simulink model "sedemsegment"  (Simulink 7.7)
settings: Solver=ode45  StartTime=0.0  StopTime=1  RelTol=1e-3
libraries: simulink x18
settings Model: Creator=RIchard  LastModifiedBy=RIchard
settings DebuggingCC: SolverPrmCheckMsg=none

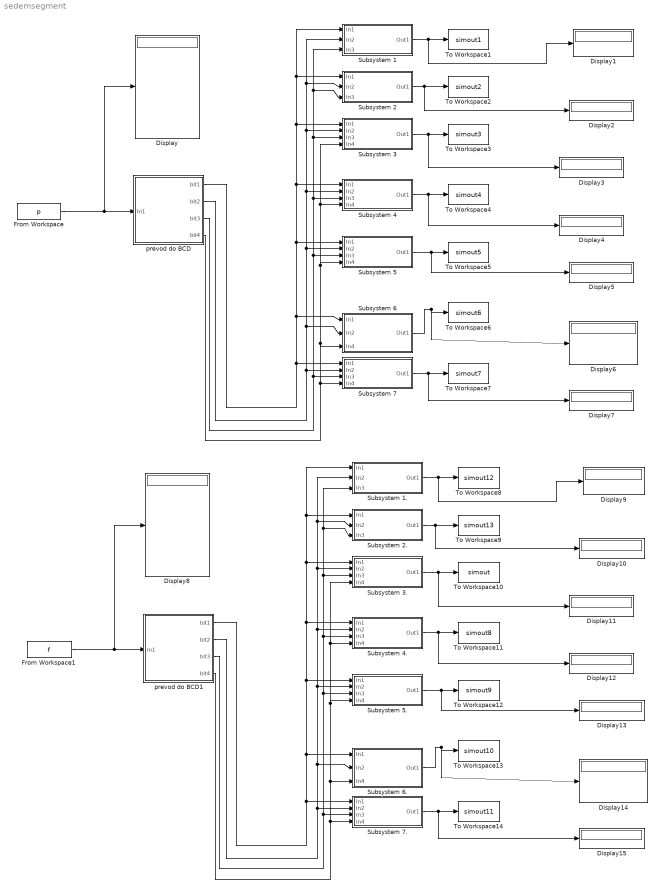
== system sedemsegment ==
  Display{,1..15} (16 alike) : Display
  From Workspace : FromWorkspace  VariableName=p  SampleTime=0
  From Workspace1 : FromWorkspace  VariableName=f  SampleTime=0
  Subsystem 1 : Subsystem  TreatAsAtomicUnit=on
  Subsystem 1. : Subsystem  TreatAsAtomicUnit=on
  Subsystem 2 : Subsystem  TreatAsAtomicUnit=on
  Subsystem 2. : Subsystem  TreatAsAtomicUnit=on
  Subsystem 3 : Subsystem  TreatAsAtomicUnit=on
  Subsystem 3. : Subsystem  TreatAsAtomicUnit=on
  Subsystem 4 : Subsystem  TreatAsAtomicUnit=on
  Subsystem 4. : Subsystem  TreatAsAtomicUnit=on
  Subsystem 5 : Subsystem  TreatAsAtomicUnit=on
  Subsystem 5. : Subsystem  TreatAsAtomicUnit=on
  Subsystem 6 : Subsystem  TreatAsAtomicUnit=on
  Subsystem 6. : Subsystem  TreatAsAtomicUnit=on
  Subsystem 7 : Subsystem  TreatAsAtomicUnit=on
  Subsystem 7. : Subsystem  TreatAsAtomicUnit=on
  To Workspace1 : ToWorkspace  VariableName=simout1  SampleTime=-1  SaveFormat=Array
  To Workspace10 : ToWorkspace  VariableName=simout  SampleTime=-1  SaveFormat=Array
  To Workspace11 : ToWorkspace  VariableName=simout8  SampleTime=-1  SaveFormat=Array
  To Workspace12 : ToWorkspace  VariableName=simout9  SampleTime=-1  SaveFormat=Array
  To Workspace13 : ToWorkspace  VariableName=simout10  SampleTime=-1  SaveFormat=Array
  To Workspace14 : ToWorkspace  VariableName=simout11  SampleTime=-1  SaveFormat=Array
  To Workspace2 : ToWorkspace  VariableName=simout2  SampleTime=-1  SaveFormat=Array
  To Workspace3 : ToWorkspace  VariableName=simout3  SampleTime=-1  SaveFormat=Array
  To Workspace4 : ToWorkspace  VariableName=simout4  SampleTime=-1  SaveFormat=Array
  To Workspace5 : ToWorkspace  VariableName=simout5  SampleTime=-1  SaveFormat=Array
  To Workspace6 : ToWorkspace  VariableName=simout6  SampleTime=-1  SaveFormat=Array
  To Workspace7 : ToWorkspace  VariableName=simout7  SampleTime=-1  SaveFormat=Array
  To Workspace8 : ToWorkspace  VariableName=simout12  SampleTime=-1  SaveFormat=Array
  To Workspace9 : ToWorkspace  VariableName=simout13  SampleTime=-1  SaveFormat=Array
  prevod do BCD : Subsystem
  prevod do BCD1 : Subsystem
  wires:
  prevod do BCD/2(bit2) -> Subsystem 7/2(In2), Subsystem 1/2(In2), Subsystem 2/2(In2), Subsystem 3/2(In2), Subsystem 4/2(In2), Subsystem 5/2(In2), Subsystem 6/2(In2)
  prevod do BCD/3(bit3) -> Subsystem 7/3(In3), Subsystem 1/3(In3), Subsystem 2/3(In3), Subsystem 3/3(In3), Subsystem 4/3(In3), Subsystem 5/3(In3)
  prevod do BCD/4(bit4) -> Subsystem 7/4(In4), Subsystem 4/4(In4), Subsystem 3/4(In4), Subsystem 5/4(In4), Subsystem 6/3(In4)
  Subsystem 1/1(Out1) -> To Workspace1/1, Display1/1
  Subsystem 2/1(Out1) -> To Workspace2/1, Display2/1
  Subsystem 3/1(Out1) -> To Workspace3/1, Display3/1
  Subsystem 4/1(Out1) -> To Workspace4/1, Display4/1
  Subsystem 5/1(Out1) -> To Workspace5/1, Display5/1
  Subsystem 7/1(Out1) -> To Workspace7/1, Display7/1
  From Workspace/1 -> prevod do BCD/1(In1), Display/1
  prevod do BCD/1(bit1) -> Subsystem 7/1(In1), Subsystem 1/1(In1), Subsystem 2/1(In1), Subsystem 3/1(In1), Subsystem 4/1(In1), Subsystem 5/1(In1), Subsystem 6/1(In1)
  Subsystem 6/1(Out1) -> To Workspace6/1, Display6/1
  prevod do BCD1/2(bit2) -> Subsystem 7./2(In2), Subsystem 1./2(In2), Subsystem 2./2(In2), Subsystem 3./2(In2), Subsystem 4./2(In2), Subsystem 5./2(In2), Subsystem 6./2(In2)
  prevod do BCD1/3(bit3) -> Subsystem 7./3(In3), Subsystem 1./3(In3), Subsystem 2./3(In3), Subsystem 3./3(In3), Subsystem 4./3(In3), Subsystem 5./3(In3)
  prevod do BCD1/4(bit4) -> Subsystem 7./4(In4), Subsystem 4./4(In4), Subsystem 3./4(In4), Subsystem 5./4(In4), Subsystem 6./3(In4)
  Subsystem 1./1(Out1) -> To Workspace8/1, Display9/1
  Subsystem 2./1(Out1) -> To Workspace9/1, Display10/1
  Subsystem 3./1(Out1) -> To Workspace10/1, Display11/1
  Subsystem 4./1(Out1) -> To Workspace11/1, Display12/1
  Subsystem 5./1(Out1) -> To Workspace12/1, Display13/1
  Subsystem 7./1(Out1) -> To Workspace14/1, Display15/1
  From Workspace1/1 -> prevod do BCD1/1(In1), Display8/1
  prevod do BCD1/1(bit1) -> Subsystem 7./1(In1), Subsystem 1./1(In1), Subsystem 2./1(In1), Subsystem 3./1(In1), Subsystem 4./1(In1), Subsystem 5./1(In1), Subsystem 6./1(In1)
  Subsystem 6./1(Out1) -> To Workspace13/1, Display14/1

== system sedemsegment/Subsystem 1 ==
  note: 1
  note: 2
  note: 3
  note: 7
  note: 8
  In1 : Inport
  In2 : Inport  Port=2
  In3 : Inport  Port=3
  Logical Operator1 : Logic  Operator=NOT  AllPortsSameDT=off  OutDataTypeStr=boolean
  Logical Operator3 : Logic  Operator=OR  AllPortsSameDT=off  OutDataTypeStr=boolean
  Logical Operator5 : Logic  AllPortsSameDT=off  OutDataTypeStr=boolean
  Out1 : Outport
  wires:
  In1/1 -> Logical Operator5/1
  In2/1 -> Logical Operator5/2
  Logical Operator1/1 -> Logical Operator3/2
  In3/1 -> Logical Operator1/1
  Logical Operator3/1 -> Out1/1
  Logical Operator5/1 -> Logical Operator3/1

== system sedemsegment/Subsystem 1. ==
  note: 1
  note: 2
  note: 3
  note: 7
  note: 8
  In1 : Inport
  In2 : Inport  Port=2
  In3 : Inport  Port=3
  Logical Operator1 : Logic  Operator=NOT  AllPortsSameDT=off  OutDataTypeStr=boolean
  Logical Operator3 : Logic  Operator=OR  AllPortsSameDT=off  OutDataTypeStr=boolean
  Logical Operator5 : Logic  AllPortsSameDT=off  OutDataTypeStr=boolean
  Out1 : Outport
  wires:
  In1/1 -> Logical Operator5/1
  In2/1 -> Logical Operator5/2
  Logical Operator1/1 -> Logical Operator3/2
  In3/1 -> Logical Operator1/1
  Logical Operator3/1 -> Out1/1
  Logical Operator5/1 -> Logical Operator3/1

== system sedemsegment/Subsystem 2 ==
  note: 1
  note: 3
  note: 4
  note: 5
  note: 6
  note: 7
  note: 8
  note: 0
  note: 9
  In1 : Inport
  In2 : Inport  Port=2
  In3 : Inport  Port=3
  Logical Operator2 : Logic  Operator=NOT  AllPortsSameDT=off  OutDataTypeStr=boolean
  Logical Operator3 : Logic  Operator=OR  Inputs=3  AllPortsSameDT=off  OutDataTypeStr=boolean
  Logical Operator6 : Logic  AllPortsSameDT=off  OutDataTypeStr=boolean
  Out1 : Outport
  wires:
  In2/1 -> Logical Operator2/1, Logical Operator6/2
  In3/1 -> Logical Operator3/3
  Logical Operator3/1 -> Out1/1
  In1/1 -> Logical Operator6/1
  Logical Operator2/1 -> Logical Operator3/1
  Logical Operator6/1 -> Logical Operator3/2

== system sedemsegment/Subsystem 2. ==
  note: 1
  note: 3
  note: 4
  note: 5
  note: 6
  note: 7
  note: 8
  note: 0
  note: 9
  In1 : Inport
  In2 : Inport  Port=2
  In3 : Inport  Port=3
  Logical Operator2 : Logic  Operator=NOT  AllPortsSameDT=off  OutDataTypeStr=boolean
  Logical Operator3 : Logic  Operator=OR  Inputs=3  AllPortsSameDT=off  OutDataTypeStr=boolean
  Logical Operator6 : Logic  AllPortsSameDT=off  OutDataTypeStr=boolean
  Out1 : Outport
  wires:
  In2/1 -> Logical Operator2/1, Logical Operator6/2
  In3/1 -> Logical Operator3/3
  Logical Operator3/1 -> Out1/1
  In1/1 -> Logical Operator6/1
  Logical Operator2/1 -> Logical Operator3/1
  Logical Operator6/1 -> Logical Operator3/2

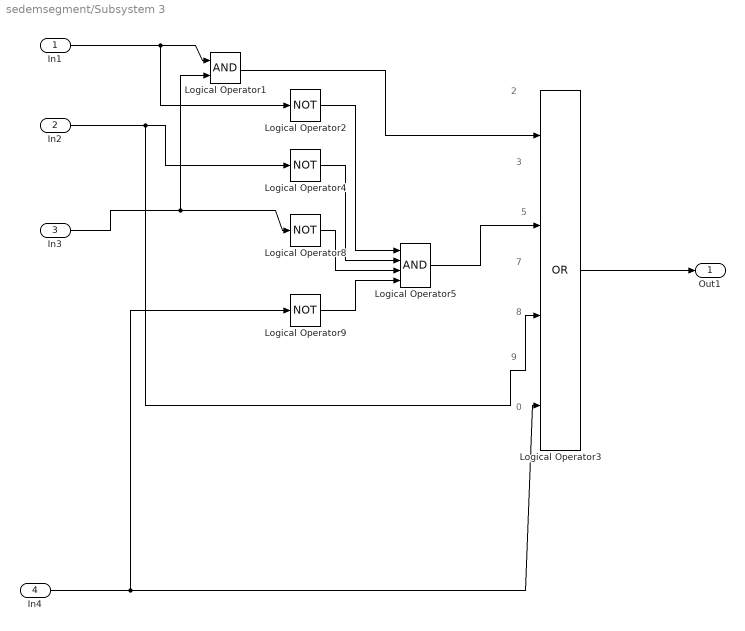
== system sedemsegment/Subsystem 3 ==
  note: 2
  note: 3
  note: 5
  note: 8
  note: 9
  note: 7
  note: 0
  In1 : Inport
  In2 : Inport  Port=2
  In3 : Inport  Port=3
  In4 : Inport  Port=4
  Logical Operator1 : Logic  AllPortsSameDT=off  OutDataTypeStr=boolean
  Logical Operator{2,4,8..9} (4 alike) : Logic  Operator=NOT  AllPortsSameDT=off  OutDataTypeStr=boolean
  Logical Operator3 : Logic  Operator=OR  Inputs=4  AllPortsSameDT=off  OutDataTypeStr=boolean
  Logical Operator5 : Logic  Inputs=4  AllPortsSameDT=off  OutDataTypeStr=boolean
  Out1 : Outport
  wires:
  In1/1 -> Logical Operator1/1, Logical Operator2/1
  In2/1 -> Logical Operator3/3, Logical Operator4/1
  In3/1 -> Logical Operator8/1, Logical Operator1/2
  In4/1 -> Logical Operator3/4, Logical Operator9/1
  Logical Operator3/1 -> Out1/1
  Logical Operator1/1 -> Logical Operator3/1
  Logical Operator2/1 -> Logical Operator5/1
  Logical Operator4/1 -> Logical Operator5/2
  Logical Operator8/1 -> Logical Operator5/3
  Logical Operator9/1 -> Logical Operator5/4
  Logical Operator5/1 -> Logical Operator3/2

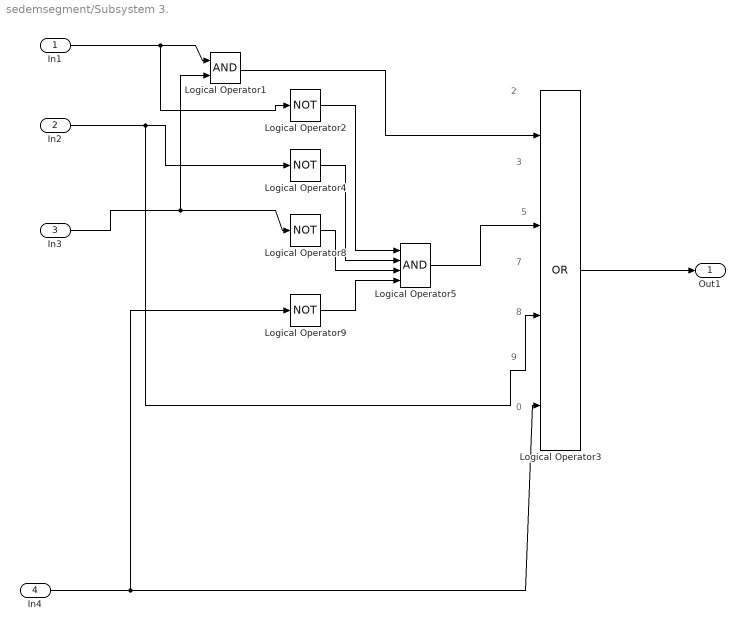
== system sedemsegment/Subsystem 3. ==
  note: 2
  note: 3
  note: 5
  note: 8
  note: 9
  note: 7
  note: 0
  In1 : Inport
  In2 : Inport  Port=2
  In3 : Inport  Port=3
  In4 : Inport  Port=4
  Logical Operator1 : Logic  AllPortsSameDT=off  OutDataTypeStr=boolean
  Logical Operator{2,4,8..9} (4 alike) : Logic  Operator=NOT  AllPortsSameDT=off  OutDataTypeStr=boolean
  Logical Operator3 : Logic  Operator=OR  Inputs=4  AllPortsSameDT=off  OutDataTypeStr=boolean
  Logical Operator5 : Logic  Inputs=4  AllPortsSameDT=off  OutDataTypeStr=boolean
  Out1 : Outport
  wires:
  In1/1 -> Logical Operator1/1, Logical Operator2/1
  In2/1 -> Logical Operator3/3, Logical Operator4/1
  In3/1 -> Logical Operator8/1, Logical Operator1/2
  In4/1 -> Logical Operator3/4, Logical Operator9/1
  Logical Operator3/1 -> Out1/1
  Logical Operator1/1 -> Logical Operator3/1
  Logical Operator2/1 -> Logical Operator5/1
  Logical Operator4/1 -> Logical Operator5/2
  Logical Operator8/1 -> Logical Operator5/3
  Logical Operator9/1 -> Logical Operator5/4
  Logical Operator5/1 -> Logical Operator3/2

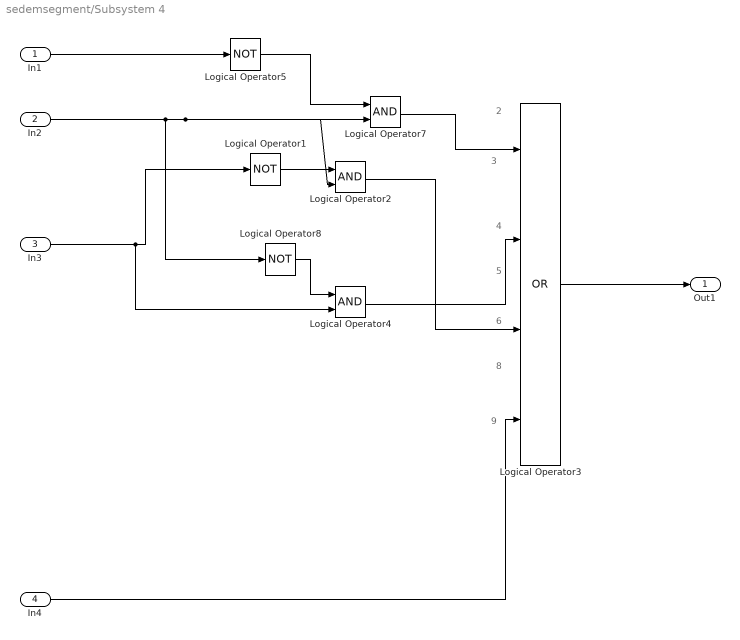
== system sedemsegment/Subsystem 4 ==
  note: 2
  note: 3
  note: 4
  note: 5
  note: 6
  note: 8
  note: 9
  In1 : Inport
  In2 : Inport  Port=2
  In3 : Inport  Port=3
  In4 : Inport  Port=4
  Logical Operator1 : Logic  Operator=NOT  AllPortsSameDT=off  OutDataTypeStr=boolean
  Logical Operator2 : Logic  AllPortsSameDT=off  OutDataTypeStr=boolean
  Logical Operator3 : Logic  Operator=OR  Inputs=4  AllPortsSameDT=off  OutDataTypeStr=boolean
  Logical Operator4 : Logic  AllPortsSameDT=off  OutDataTypeStr=boolean
  Logical Operator5 : Logic  Operator=NOT  AllPortsSameDT=off  OutDataTypeStr=boolean
  Logical Operator7 : Logic  AllPortsSameDT=off  OutDataTypeStr=boolean
  Logical Operator8 : Logic  Operator=NOT  AllPortsSameDT=off  OutDataTypeStr=boolean
  Out1 : Outport
  wires:
  Logical Operator3/1 -> Out1/1
  In3/1 -> Logical Operator1/1, Logical Operator4/2
  In2/1 -> Logical Operator2/2, Logical Operator7/2, Logical Operator8/1
  Logical Operator1/1 -> Logical Operator2/1
  In4/1 -> Logical Operator3/4
  Logical Operator2/1 -> Logical Operator3/3
  In1/1 -> Logical Operator5/1
  Logical Operator7/1 -> Logical Operator3/1
  Logical Operator5/1 -> Logical Operator7/1
  Logical Operator8/1 -> Logical Operator4/1
  Logical Operator4/1 -> Logical Operator3/2

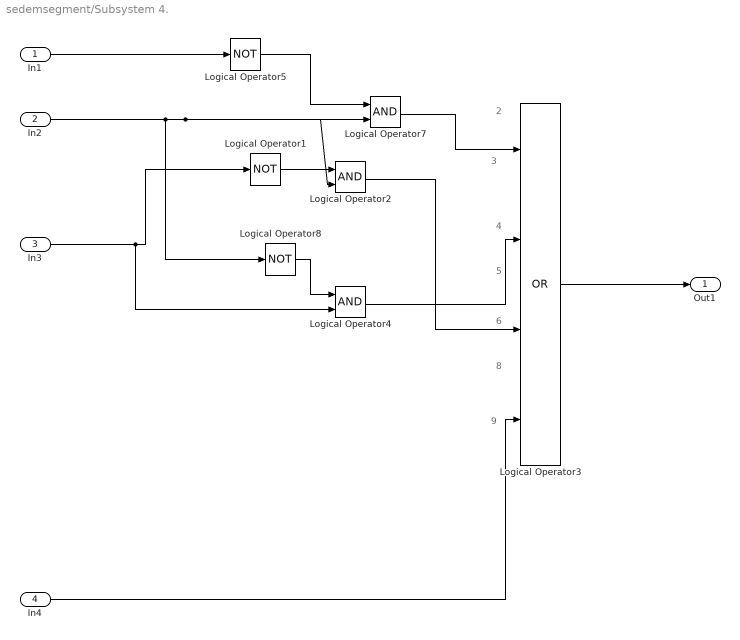
== system sedemsegment/Subsystem 4. ==
  note: 2
  note: 3
  note: 4
  note: 5
  note: 6
  note: 8
  note: 9
  In1 : Inport
  In2 : Inport  Port=2
  In3 : Inport  Port=3
  In4 : Inport  Port=4
  Logical Operator1 : Logic  Operator=NOT  AllPortsSameDT=off  OutDataTypeStr=boolean
  Logical Operator2 : Logic  AllPortsSameDT=off  OutDataTypeStr=boolean
  Logical Operator3 : Logic  Operator=OR  Inputs=4  AllPortsSameDT=off  OutDataTypeStr=boolean
  Logical Operator4 : Logic  AllPortsSameDT=off  OutDataTypeStr=boolean
  Logical Operator5 : Logic  Operator=NOT  AllPortsSameDT=off  OutDataTypeStr=boolean
  Logical Operator7 : Logic  AllPortsSameDT=off  OutDataTypeStr=boolean
  Logical Operator8 : Logic  Operator=NOT  AllPortsSameDT=off  OutDataTypeStr=boolean
  Out1 : Outport
  wires:
  Logical Operator3/1 -> Out1/1
  In3/1 -> Logical Operator1/1, Logical Operator4/2
  In2/1 -> Logical Operator2/2, Logical Operator7/2, Logical Operator8/1
  Logical Operator1/1 -> Logical Operator2/1
  In4/1 -> Logical Operator3/4
  Logical Operator2/1 -> Logical Operator3/3
  In1/1 -> Logical Operator5/1
  Logical Operator7/1 -> Logical Operator3/1
  Logical Operator5/1 -> Logical Operator7/1
  Logical Operator8/1 -> Logical Operator4/1
  Logical Operator4/1 -> Logical Operator3/2

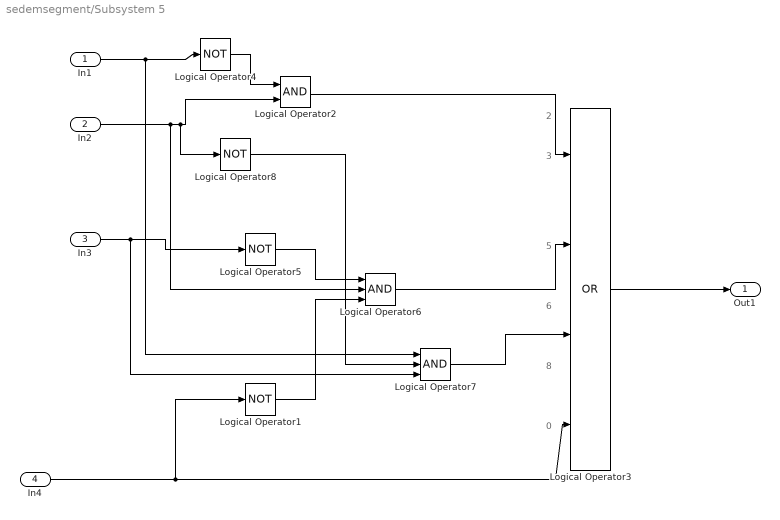
== system sedemsegment/Subsystem 5 ==
  note: 2
  note: 3
  note: 5
  note: 6
  note: 8
  note: 0
  In1 : Inport
  In2 : Inport  Port=2
  In3 : Inport  Port=3
  In4 : Inport  Port=4
  Logical Operator{1,4..5,8} (4 alike) : Logic  Operator=NOT  AllPortsSameDT=off  OutDataTypeStr=boolean
  Logical Operator2 : Logic  AllPortsSameDT=off  OutDataTypeStr=boolean
  Logical Operator3 : Logic  Operator=OR  Inputs=4  AllPortsSameDT=off  OutDataTypeStr=boolean
  Logical Operator6 : Logic  Inputs=3  AllPortsSameDT=off  OutDataTypeStr=boolean
  Logical Operator7 : Logic  Inputs=3  AllPortsSameDT=off  OutDataTypeStr=boolean
  Out1 : Outport
  wires:
  Logical Operator3/1 -> Out1/1
  In4/1 -> Logical Operator3/4, Logical Operator1/1
  In1/1 -> Logical Operator4/1, Logical Operator7/1
  Logical Operator4/1 -> Logical Operator2/1
  In2/1 -> Logical Operator6/2, Logical Operator2/2, Logical Operator8/1
  Logical Operator2/1 -> Logical Operator3/1
  In3/1 -> Logical Operator5/1, Logical Operator7/3
  Logical Operator5/1 -> Logical Operator6/1
  Logical Operator1/1 -> Logical Operator6/3
  Logical Operator6/1 -> Logical Operator3/2
  Logical Operator7/1 -> Logical Operator3/3
  Logical Operator8/1 -> Logical Operator7/2

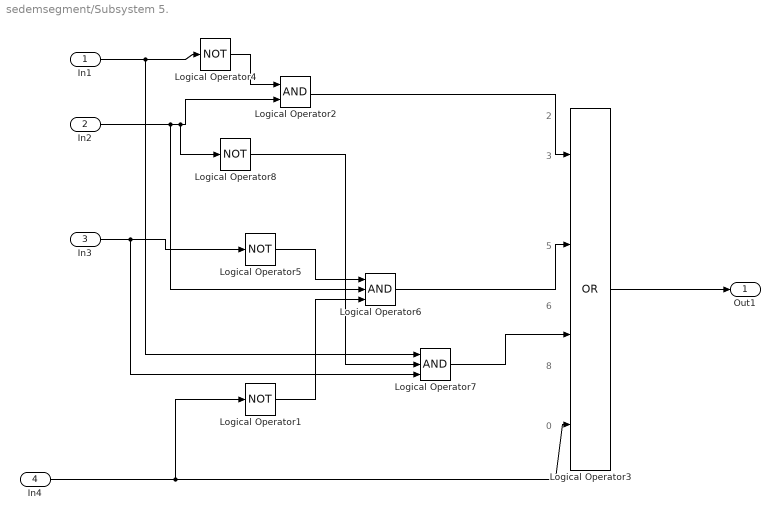
== system sedemsegment/Subsystem 5. ==
  note: 2
  note: 3
  note: 5
  note: 6
  note: 8
  note: 0
  In1 : Inport
  In2 : Inport  Port=2
  In3 : Inport  Port=3
  In4 : Inport  Port=4
  Logical Operator{1,4..5,8} (4 alike) : Logic  Operator=NOT  AllPortsSameDT=off  OutDataTypeStr=boolean
  Logical Operator2 : Logic  AllPortsSameDT=off  OutDataTypeStr=boolean
  Logical Operator3 : Logic  Operator=OR  Inputs=4  AllPortsSameDT=off  OutDataTypeStr=boolean
  Logical Operator6 : Logic  Inputs=3  AllPortsSameDT=off  OutDataTypeStr=boolean
  Logical Operator7 : Logic  Inputs=3  AllPortsSameDT=off  OutDataTypeStr=boolean
  Out1 : Outport
  wires:
  Logical Operator3/1 -> Out1/1
  In4/1 -> Logical Operator3/4, Logical Operator1/1
  In1/1 -> Logical Operator4/1, Logical Operator7/1
  Logical Operator4/1 -> Logical Operator2/1
  In2/1 -> Logical Operator6/2, Logical Operator2/2, Logical Operator8/1
  Logical Operator2/1 -> Logical Operator3/1
  In3/1 -> Logical Operator5/1, Logical Operator7/3
  Logical Operator5/1 -> Logical Operator6/1
  Logical Operator1/1 -> Logical Operator6/3
  Logical Operator6/1 -> Logical Operator3/2
  Logical Operator7/1 -> Logical Operator3/3
  Logical Operator8/1 -> Logical Operator7/2

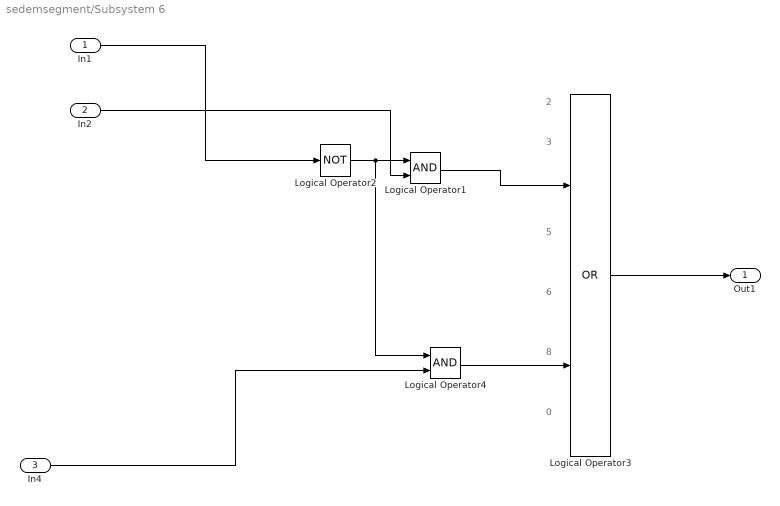
== system sedemsegment/Subsystem 6 ==
  note: 2
  note: 3
  note: 5
  note: 6
  note: 8
  note: 0
  In1 : Inport
  In2 : Inport  Port=2
  In4 : Inport  Port=3
  Logical Operator1 : Logic  AllPortsSameDT=off  OutDataTypeStr=boolean
  Logical Operator2 : Logic  Operator=NOT  AllPortsSameDT=off  OutDataTypeStr=boolean
  Logical Operator3 : Logic  Operator=OR  AllPortsSameDT=off  OutDataTypeStr=boolean
  Logical Operator4 : Logic  AllPortsSameDT=off  OutDataTypeStr=boolean
  Out1 : Outport
  wires:
  Logical Operator3/1 -> Out1/1
  In1/1 -> Logical Operator2/1
  Logical Operator2/1 -> Logical Operator1/1, Logical Operator4/1
  Logical Operator4/1 -> Logical Operator3/2
  In4/1 -> Logical Operator4/2
  Logical Operator1/1 -> Logical Operator3/1
  In2/1 -> Logical Operator1/2

== system sedemsegment/Subsystem 6. ==
  note: 2
  note: 3
  note: 5
  note: 6
  note: 8
  note: 0
  In1 : Inport
  In2 : Inport  Port=2
  In4 : Inport  Port=3
  Logical Operator1 : Logic  AllPortsSameDT=off  OutDataTypeStr=boolean
  Logical Operator2 : Logic  Operator=NOT  AllPortsSameDT=off  OutDataTypeStr=boolean
  Logical Operator3 : Logic  Operator=OR  AllPortsSameDT=off  OutDataTypeStr=boolean
  Logical Operator4 : Logic  AllPortsSameDT=off  OutDataTypeStr=boolean
  Out1 : Outport
  wires:
  Logical Operator3/1 -> Out1/1
  In1/1 -> Logical Operator2/1
  Logical Operator2/1 -> Logical Operator1/1, Logical Operator4/1
  Logical Operator4/1 -> Logical Operator3/2
  In4/1 -> Logical Operator4/2
  Logical Operator1/1 -> Logical Operator3/1
  In2/1 -> Logical Operator1/2

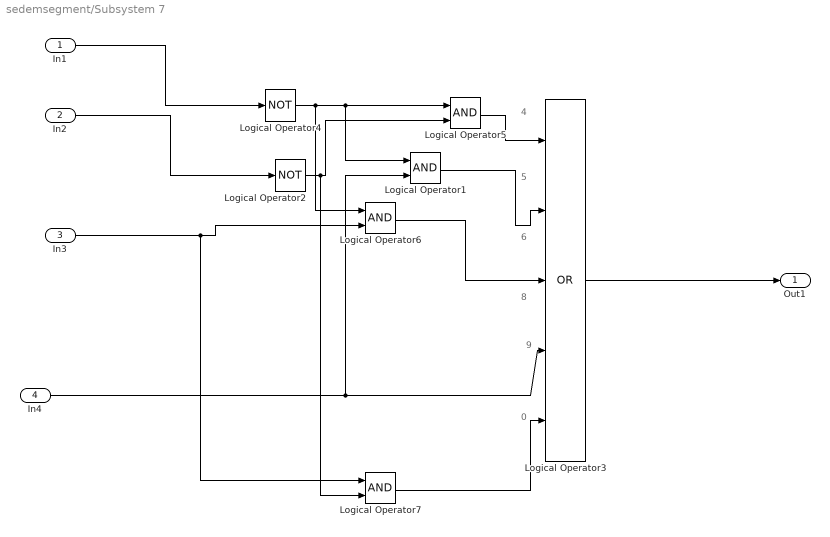
== system sedemsegment/Subsystem 7 ==
  note: 4
  note: 5
  note: 6
  note: 8
  note: 9
  note: 0
  In1 : Inport
  In2 : Inport  Port=2
  In3 : Inport  Port=3
  In4 : Inport  Port=4
  Logical Operator{1,5..7} (4 alike) : Logic  AllPortsSameDT=off  OutDataTypeStr=boolean
  Logical Operator2 : Logic  Operator=NOT  AllPortsSameDT=off  OutDataTypeStr=boolean
  Logical Operator3 : Logic  Operator=OR  Inputs=5  AllPortsSameDT=off  OutDataTypeStr=boolean
  Logical Operator4 : Logic  Operator=NOT  AllPortsSameDT=off  OutDataTypeStr=boolean
  Out1 : Outport
  wires:
  Logical Operator3/1 -> Out1/1
  Logical Operator2/1 -> Logical Operator5/2, Logical Operator7/2
  In4/1 -> Logical Operator3/4, Logical Operator1/2
  In2/1 -> Logical Operator2/1
  In3/1 -> Logical Operator6/2, Logical Operator7/1
  Logical Operator6/1 -> Logical Operator3/3
  Logical Operator1/1 -> Logical Operator3/2
  In1/1 -> Logical Operator4/1
  Logical Operator4/1 -> Logical Operator1/1, Logical Operator5/1, Logical Operator6/1
  Logical Operator5/1 -> Logical Operator3/1
  Logical Operator7/1 -> Logical Operator3/5

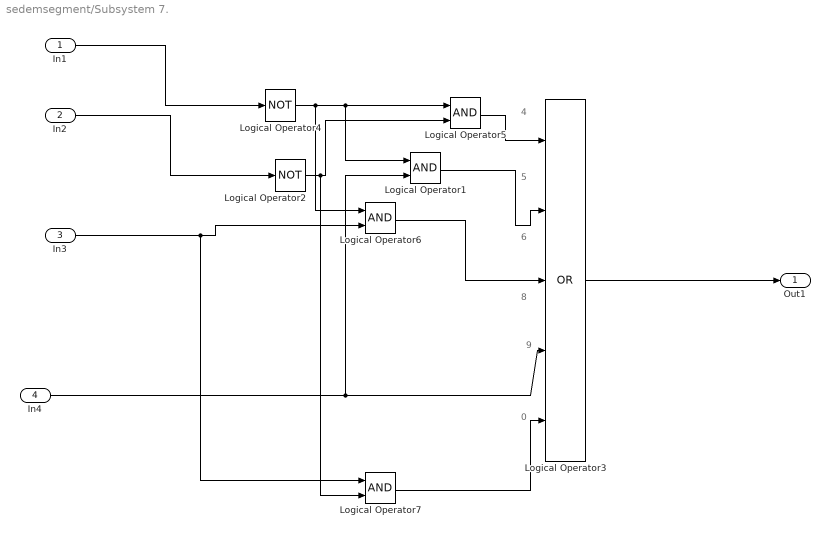
== system sedemsegment/Subsystem 7. ==
  note: 4
  note: 5
  note: 6
  note: 8
  note: 9
  note: 0
  In1 : Inport
  In2 : Inport  Port=2
  In3 : Inport  Port=3
  In4 : Inport  Port=4
  Logical Operator{1,5..7} (4 alike) : Logic  AllPortsSameDT=off  OutDataTypeStr=boolean
  Logical Operator2 : Logic  Operator=NOT  AllPortsSameDT=off  OutDataTypeStr=boolean
  Logical Operator3 : Logic  Operator=OR  Inputs=5  AllPortsSameDT=off  OutDataTypeStr=boolean
  Logical Operator4 : Logic  Operator=NOT  AllPortsSameDT=off  OutDataTypeStr=boolean
  Out1 : Outport
  wires:
  Logical Operator3/1 -> Out1/1
  Logical Operator2/1 -> Logical Operator5/2, Logical Operator7/2
  In4/1 -> Logical Operator3/4, Logical Operator1/2
  In2/1 -> Logical Operator2/1
  In3/1 -> Logical Operator6/2, Logical Operator7/1
  Logical Operator6/1 -> Logical Operator3/3
  Logical Operator1/1 -> Logical Operator3/2
  In1/1 -> Logical Operator4/1
  Logical Operator4/1 -> Logical Operator1/1, Logical Operator5/1, Logical Operator6/1
  Logical Operator5/1 -> Logical Operator3/1
  Logical Operator7/1 -> Logical Operator3/5

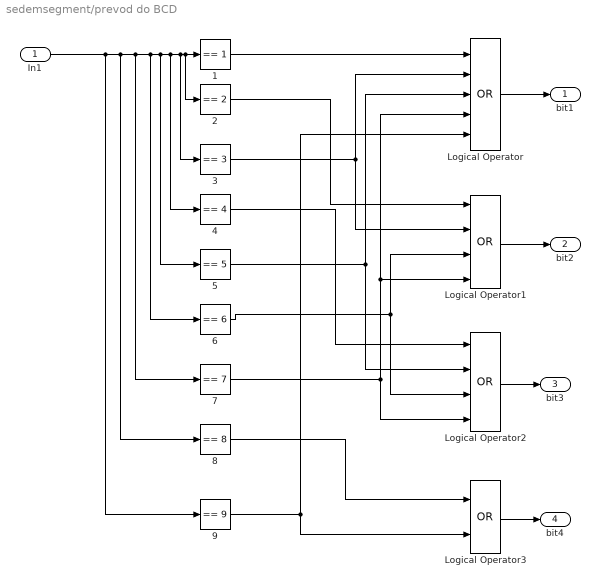
== system sedemsegment/prevod do BCD ==
  In1 : Inport
  "  5" : simulink/Logic and Bit Operations/Compare To Constant  SystemSampleTime=-1  relop===  const=5  LogicOutDataTypeMode=uint8
  " 1" : simulink/Logic and Bit Operations/Compare To Constant  SystemSampleTime=-1  relop===  const=1  LogicOutDataTypeMode=uint8
  " 2" : simulink/Logic and Bit Operations/Compare To Constant  SystemSampleTime=-1  relop===  const=2  LogicOutDataTypeMode=uint8
  " 3" : simulink/Logic and Bit Operations/Compare To Constant  SystemSampleTime=-1  relop===  const=3  LogicOutDataTypeMode=uint8
  " 4" : simulink/Logic and Bit Operations/Compare To Constant  SystemSampleTime=-1  relop===  const=4  LogicOutDataTypeMode=uint8
  "6    " : simulink/Logic and Bit Operations/Compare To Constant  SystemSampleTime=-1  relop===  const=6  LogicOutDataTypeMode=uint8
  "7    " : simulink/Logic and Bit Operations/Compare To Constant  SystemSampleTime=-1  relop===  const=7  LogicOutDataTypeMode=uint8
  "8  " : simulink/Logic and Bit Operations/Compare To Constant  SystemSampleTime=-1  relop===  const=8  LogicOutDataTypeMode=uint8
  "9 " : simulink/Logic and Bit Operations/Compare To Constant  SystemSampleTime=-1  relop===  const=9  LogicOutDataTypeMode=uint8
  Logical Operator : Logic  Operator=OR  Inputs=5  AllPortsSameDT=off  OutDataTypeStr=boolean
  Logical Operator1 : Logic  Operator=OR  Inputs=4  AllPortsSameDT=off  OutDataTypeStr=boolean
  Logical Operator2 : Logic  Operator=OR  Inputs=4  AllPortsSameDT=off  OutDataTypeStr=boolean
  Logical Operator3 : Logic  Operator=OR  AllPortsSameDT=off  OutDataTypeStr=boolean
  bit1 : Outport
  bit2 : Outport  Port=2
  bit3 : Outport  Port=3
  bit4 : Outport  Port=4
  wires:
  In1/1 -> " 1"/1, " 2"/1, " 3"/1, " 4"/1, "  5"/1, "6    "/1, "7    "/1, "8  "/1, "9 "/1
  " 1"/1 -> Logical Operator/1
  " 2"/1 -> Logical Operator1/1
  " 3"/1 -> Logical Operator/2, Logical Operator1/2
  " 4"/1 -> Logical Operator2/1
  "  5"/1 -> Logical Operator/3, Logical Operator2/2
  "6    "/1 -> Logical Operator1/3, Logical Operator2/3
  "7    "/1 -> Logical Operator2/4, Logical Operator1/4, Logical Operator/4
  "8  "/1 -> Logical Operator3/1
  "9 "/1 -> Logical Operator3/2, Logical Operator/5
  Logical Operator/1 -> bit1/1
  Logical Operator1/1 -> bit2/1
  Logical Operator2/1 -> bit3/1
  Logical Operator3/1 -> bit4/1

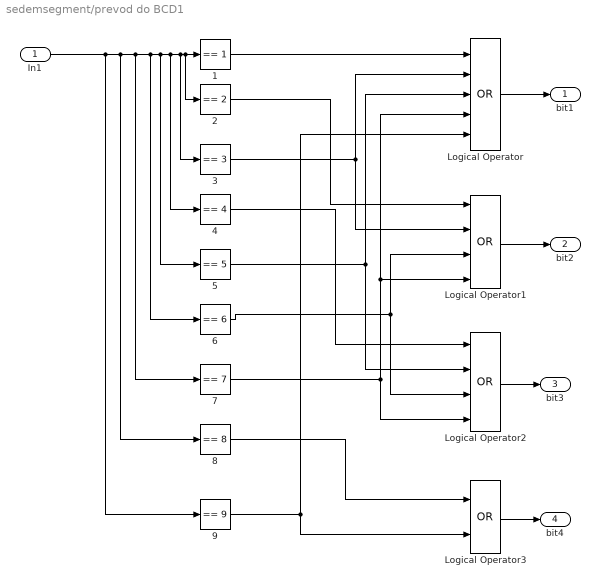
== system sedemsegment/prevod do BCD1 ==
  In1 : Inport
  "  5" : simulink/Logic and Bit Operations/Compare To Constant  SystemSampleTime=-1  relop===  const=5  LogicOutDataTypeMode=uint8
  " 1" : simulink/Logic and Bit Operations/Compare To Constant  SystemSampleTime=-1  relop===  const=1  LogicOutDataTypeMode=uint8
  " 2" : simulink/Logic and Bit Operations/Compare To Constant  SystemSampleTime=-1  relop===  const=2  LogicOutDataTypeMode=uint8
  " 3" : simulink/Logic and Bit Operations/Compare To Constant  SystemSampleTime=-1  relop===  const=3  LogicOutDataTypeMode=uint8
  " 4" : simulink/Logic and Bit Operations/Compare To Constant  SystemSampleTime=-1  relop===  const=4  LogicOutDataTypeMode=uint8
  "6    " : simulink/Logic and Bit Operations/Compare To Constant  SystemSampleTime=-1  relop===  const=6  LogicOutDataTypeMode=uint8
  "7    " : simulink/Logic and Bit Operations/Compare To Constant  SystemSampleTime=-1  relop===  const=7  LogicOutDataTypeMode=uint8
  "8  " : simulink/Logic and Bit Operations/Compare To Constant  SystemSampleTime=-1  relop===  const=8  LogicOutDataTypeMode=uint8
  "9 " : simulink/Logic and Bit Operations/Compare To Constant  SystemSampleTime=-1  relop===  const=9  LogicOutDataTypeMode=uint8
  Logical Operator : Logic  Operator=OR  Inputs=5  AllPortsSameDT=off  OutDataTypeStr=boolean
  Logical Operator1 : Logic  Operator=OR  Inputs=4  AllPortsSameDT=off  OutDataTypeStr=boolean
  Logical Operator2 : Logic  Operator=OR  Inputs=4  AllPortsSameDT=off  OutDataTypeStr=boolean
  Logical Operator3 : Logic  Operator=OR  AllPortsSameDT=off  OutDataTypeStr=boolean
  bit1 : Outport
  bit2 : Outport  Port=2
  bit3 : Outport  Port=3
  bit4 : Outport  Port=4
  wires:
  In1/1 -> " 1"/1, " 2"/1, " 3"/1, " 4"/1, "  5"/1, "6    "/1, "7    "/1, "8  "/1, "9 "/1
  " 1"/1 -> Logical Operator/1
  " 2"/1 -> Logical Operator1/1
  " 3"/1 -> Logical Operator/2, Logical Operator1/2
  " 4"/1 -> Logical Operator2/1
  "  5"/1 -> Logical Operator/3, Logical Operator2/2
  "6    "/1 -> Logical Operator1/3, Logical Operator2/3
  "7    "/1 -> Logical Operator2/4, Logical Operator1/4, Logical Operator/4
  "8  "/1 -> Logical Operator3/1
  "9 "/1 -> Logical Operator3/2, Logical Operator/5
  Logical Operator/1 -> bit1/1
  Logical Operator1/1 -> bit2/1
  Logical Operator2/1 -> bit3/1
  Logical Operator3/1 -> bit4/1
